simulink model "cart_pendulum_staged_comparison"  (R2018b)
settings: Solver=ode45  StartTime=0.0  StopTime=20  MaxStep=.001  RelTol=1e-8  AbsTol=1e-10
model workspace (MAT data in the model file):
  Ad = [0.884694915571  0.00188314730074  1.9215788783e-06; -2.27514939191  0.997683753616  0.00199844203344; -15.0651784059  -0.0153726310264  0.99998964827]
  Bd = [0.115305084429  1.9215788783e-06; 2.27514939191  0.00199844203344; 15.0651784059  -1.0351730262e-05]
  I = 0.006
  K = [-10 -10.945744415 59.5938842387 10.3435378998]
  M = 0.5
  b = 0.1
  disturbance_ts = [0  0; 8  1; 8.1  0; 20  0]
  g = 9.8
  l = 0.3
  m = 0.2
  z0 = [0; 0; 0.0872664625997; 0]
settings Model: Creator=volka  LastModifiedBy=volka
settings DataIOCC: ReturnWorkspaceOutputs=on

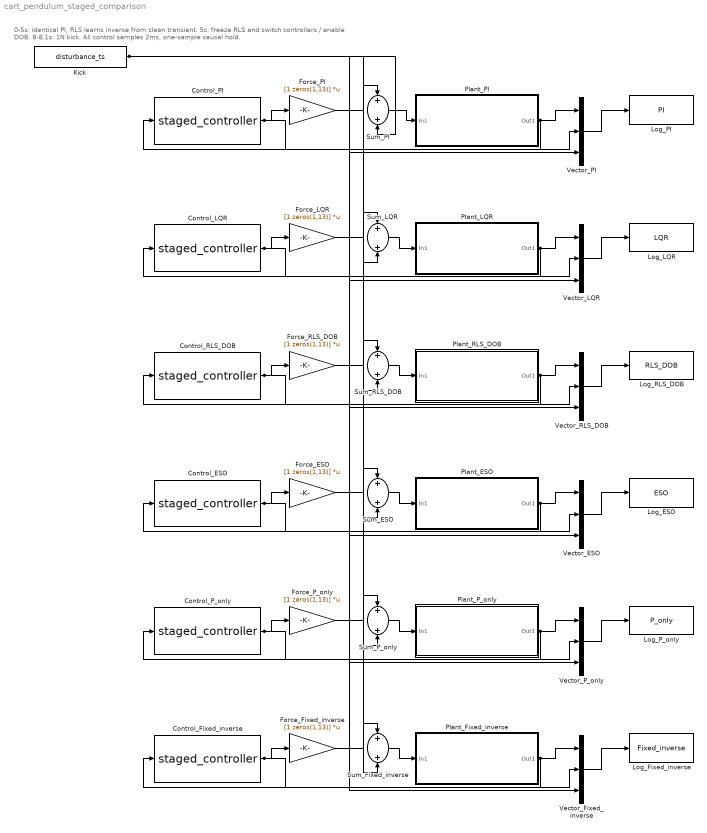
== system cart_pendulum_staged_comparison ==
  note: 0-5s: identical PI, RLS learns inverse from clean transient. 5s: freeze RLS and switch controllers / enable DOB. 8-8.1s: 1N kick. All control samples 2ms, one-sample causal hold.
  Control_ESO : S-Function  FunctionName=staged_controller  Parameters=4,K,Ad,Bd  SFunctionDeploymentMode=off  EnableBusSupport=off
  Control_Fixed_inverse : S-Function  FunctionName=staged_controller  Parameters=6,K,Ad,Bd  SFunctionDeploymentMode=off  EnableBusSupport=off
  Control_LQR : S-Function  FunctionName=staged_controller  Parameters=2,K,Ad,Bd  SFunctionDeploymentMode=off  EnableBusSupport=off
  Control_PI : S-Function  FunctionName=staged_controller  Parameters=1,K,Ad,Bd  SFunctionDeploymentMode=off  EnableBusSupport=off
  Control_P_only : S-Function  FunctionName=staged_controller  Parameters=5,K,Ad,Bd  SFunctionDeploymentMode=off  EnableBusSupport=off
  Control_RLS_DOB : S-Function  FunctionName=staged_controller  Parameters=3,K,Ad,Bd  SFunctionDeploymentMode=off  EnableBusSupport=off
  Force_ESO : Gain  Gain=[1 zeros(1,13)]  Multiplication=Matrix(K*u)
  Force_Fixed_inverse : Gain  Gain=[1 zeros(1,13)]  Multiplication=Matrix(K*u)
  Force_LQR : Gain  Gain=[1 zeros(1,13)]  Multiplication=Matrix(K*u)
  Force_PI : Gain  Gain=[1 zeros(1,13)]  Multiplication=Matrix(K*u)
  Force_P_only : Gain  Gain=[1 zeros(1,13)]  Multiplication=Matrix(K*u)
  Force_RLS_DOB : Gain  Gain=[1 zeros(1,13)]  Multiplication=Matrix(K*u)
  Kick : FromWorkspace  VariableName=disturbance_ts  SampleTime=0  Interpolate=off  OutputAfterFinalValue=Holding final value
  Log_ESO : ToWorkspace  VariableName=ESO  SaveFormat=Structure With Time  SampleTime=-1
  Log_Fixed_inverse : ToWorkspace  VariableName=Fixed_inverse  SaveFormat=Structure With Time  SampleTime=-1
  Log_LQR : ToWorkspace  VariableName=LQR  SaveFormat=Structure With Time  SampleTime=-1
  Log_PI : ToWorkspace  VariableName=PI  SaveFormat=Structure With Time  SampleTime=-1
  Log_P_only : ToWorkspace  VariableName=P_only  SaveFormat=Structure With Time  SampleTime=-1
  Log_RLS_DOB : ToWorkspace  VariableName=RLS_DOB  SaveFormat=Structure With Time  SampleTime=-1
  Plant_ESO : Subsystem
  Plant_Fixed_inverse : Subsystem
  Plant_LQR : Subsystem
  Plant_PI : Subsystem
  Plant_P_only : Subsystem
  Plant_RLS_DOB : Subsystem
  Sum_ESO : Sum
  Sum_Fixed_inverse : Sum
  Sum_LQR : Sum
  Sum_PI : Sum
  Sum_P_only : Sum
  Sum_RLS_DOB : Sum
  Vector_ESO : Mux  Inputs=3
  Vector_Fixed_inverse : Mux  Inputs=3
  Vector_LQR : Mux  Inputs=3
  Vector_PI : Mux  Inputs=3
  Vector_P_only : Mux  Inputs=3
  Vector_RLS_DOB : Mux  Inputs=3
  wires:
  Plant_PI/1(Out1) -> Control_PI/1, Vector_PI/1
  Control_PI/1 -> Force_PI/1, Vector_PI/2
  Force_PI/1 -> Sum_PI/1
  Kick/1 -> Sum_PI/2, Vector_PI/3, Sum_LQR/2, Vector_LQR/3, Sum_RLS_DOB/2, Vector_RLS_DOB/3, Sum_ESO/2, Vector_ESO/3, Sum_P_only/2, Vector_P_only/3, Sum_Fixed_inverse/2, Vector_Fixed_inverse/3
  Sum_PI/1 -> Plant_PI/1(In1)
  Vector_PI/1 -> Log_PI/1
  Plant_LQR/1(Out1) -> Control_LQR/1, Vector_LQR/1
  Control_LQR/1 -> Force_LQR/1, Vector_LQR/2
  Force_LQR/1 -> Sum_LQR/1
  Sum_LQR/1 -> Plant_LQR/1(In1)
  Vector_LQR/1 -> Log_LQR/1
  Plant_RLS_DOB/1(Out1) -> Control_RLS_DOB/1, Vector_RLS_DOB/1
  Control_RLS_DOB/1 -> Force_RLS_DOB/1, Vector_RLS_DOB/2
  Force_RLS_DOB/1 -> Sum_RLS_DOB/1
  Sum_RLS_DOB/1 -> Plant_RLS_DOB/1(In1)
  Vector_RLS_DOB/1 -> Log_RLS_DOB/1
  Plant_ESO/1(Out1) -> Control_ESO/1, Vector_ESO/1
  Control_ESO/1 -> Force_ESO/1, Vector_ESO/2
  Force_ESO/1 -> Sum_ESO/1
  Sum_ESO/1 -> Plant_ESO/1(In1)
  Vector_ESO/1 -> Log_ESO/1
  Plant_P_only/1(Out1) -> Control_P_only/1, Vector_P_only/1
  Control_P_only/1 -> Force_P_only/1, Vector_P_only/2
  Force_P_only/1 -> Sum_P_only/1
  Sum_P_only/1 -> Plant_P_only/1(In1)
  Vector_P_only/1 -> Log_P_only/1
  Plant_Fixed_inverse/1(Out1) -> Control_Fixed_inverse/1, Vector_Fixed_inverse/1
  Control_Fixed_inverse/1 -> Force_Fixed_inverse/1, Vector_Fixed_inverse/2
  Force_Fixed_inverse/1 -> Sum_Fixed_inverse/1
  Sum_Fixed_inverse/1 -> Plant_Fixed_inverse/1(In1)
  Vector_Fixed_inverse/1 -> Log_Fixed_inverse/1

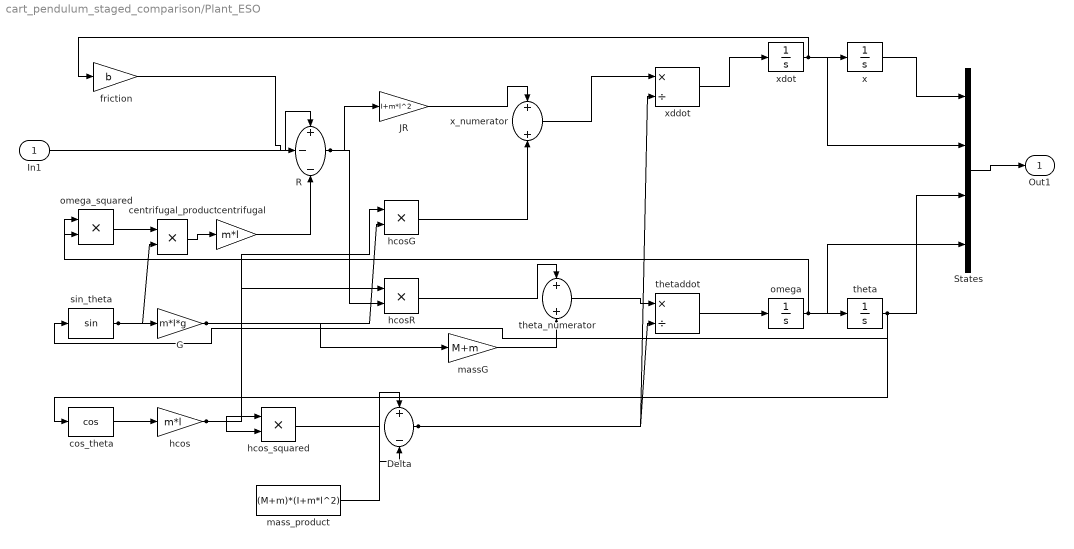
== system cart_pendulum_staged_comparison/Plant_ESO ==
  In1 : Inport
  Delta : Sum  Inputs=+-
  G : Gain  Gain=m*l*g
  JR : Gain  Gain=I+m*l^2
  R : Sum  Inputs=+--
  States : Mux
  centrifugal : Gain  Gain=m*l
  centrifugal_product : Product  Inputs=**
  cos_theta : Trigonometry  Operator=cos
  friction : Gain  Gain=b
  hcos : Gain  Gain=m*l
  hcosG : Product  Inputs=**
  hcosR : Product  Inputs=**
  hcos_squared : Product  Inputs=**
  massG : Gain  Gain=M+m
  mass_product : Constant  Value=(M+m)*(I+m*l^2)
  omega : Integrator  InitialCondition=z0(4)
  omega_squared : Product  Inputs=**
  sin_theta : Trigonometry
  theta : Integrator  InitialCondition=z0(3)
  theta_numerator : Sum
  thetaddot : Product  Inputs=*/
  x : Integrator  InitialCondition=z0(1)
  x_numerator : Sum
  xddot : Product  Inputs=*/
  xdot : Integrator  InitialCondition=z0(2)
  Out1 : Outport
  wires:
  States/1 -> Out1/1
  x/1 -> States/1
  thetaddot/1 -> omega/1
  xddot/1 -> xdot/1
  theta_numerator/1 -> thetaddot/1
  Delta/1 -> thetaddot/2, xddot/2
  x_numerator/1 -> xddot/1
  massG/1 -> theta_numerator/2
  hcosR/1 -> theta_numerator/1
  hcosG/1 -> x_numerator/2
  JR/1 -> x_numerator/1
  G/1 -> massG/1, hcosG/2
  R/1 -> hcosR/2, JR/1
  hcos_squared/1 -> Delta/2
  mass_product/1 -> Delta/1
  hcos/1 -> hcosR/1, hcosG/1, hcos_squared/2, hcos_squared/1
  cos_theta/1 -> hcos/1
  centrifugal/1 -> R/3
  centrifugal_product/1 -> centrifugal/1
  sin_theta/1 -> G/1, centrifugal_product/2
  theta/1 -> States/3, cos_theta/1, sin_theta/1
  omega_squared/1 -> centrifugal_product/1
  omega/1 -> States/4, theta/1, omega_squared/2, omega_squared/1
  friction/1 -> R/2
  xdot/1 -> States/2, x/1, friction/1
  In1/1 -> R/1

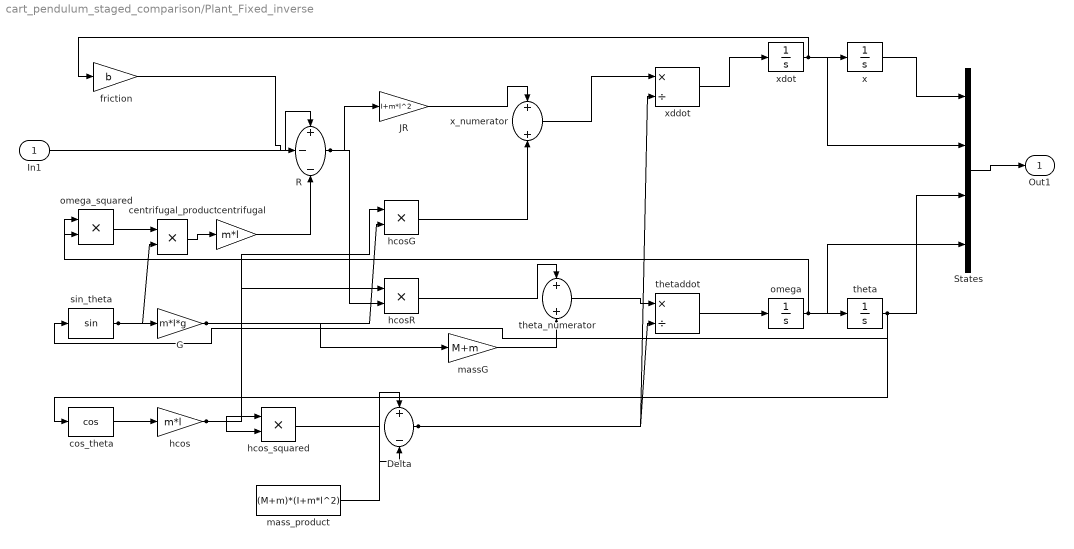
== system cart_pendulum_staged_comparison/Plant_Fixed_inverse ==
  In1 : Inport
  Delta : Sum  Inputs=+-
  G : Gain  Gain=m*l*g
  JR : Gain  Gain=I+m*l^2
  R : Sum  Inputs=+--
  States : Mux
  centrifugal : Gain  Gain=m*l
  centrifugal_product : Product  Inputs=**
  cos_theta : Trigonometry  Operator=cos
  friction : Gain  Gain=b
  hcos : Gain  Gain=m*l
  hcosG : Product  Inputs=**
  hcosR : Product  Inputs=**
  hcos_squared : Product  Inputs=**
  massG : Gain  Gain=M+m
  mass_product : Constant  Value=(M+m)*(I+m*l^2)
  omega : Integrator  InitialCondition=z0(4)
  omega_squared : Product  Inputs=**
  sin_theta : Trigonometry
  theta : Integrator  InitialCondition=z0(3)
  theta_numerator : Sum
  thetaddot : Product  Inputs=*/
  x : Integrator  InitialCondition=z0(1)
  x_numerator : Sum
  xddot : Product  Inputs=*/
  xdot : Integrator  InitialCondition=z0(2)
  Out1 : Outport
  wires:
  States/1 -> Out1/1
  x/1 -> States/1
  thetaddot/1 -> omega/1
  xddot/1 -> xdot/1
  theta_numerator/1 -> thetaddot/1
  Delta/1 -> thetaddot/2, xddot/2
  x_numerator/1 -> xddot/1
  massG/1 -> theta_numerator/2
  hcosR/1 -> theta_numerator/1
  hcosG/1 -> x_numerator/2
  JR/1 -> x_numerator/1
  G/1 -> massG/1, hcosG/2
  R/1 -> hcosR/2, JR/1
  hcos_squared/1 -> Delta/2
  mass_product/1 -> Delta/1
  hcos/1 -> hcosR/1, hcosG/1, hcos_squared/2, hcos_squared/1
  cos_theta/1 -> hcos/1
  centrifugal/1 -> R/3
  centrifugal_product/1 -> centrifugal/1
  sin_theta/1 -> G/1, centrifugal_product/2
  theta/1 -> States/3, cos_theta/1, sin_theta/1
  omega_squared/1 -> centrifugal_product/1
  omega/1 -> States/4, theta/1, omega_squared/2, omega_squared/1
  friction/1 -> R/2
  xdot/1 -> States/2, x/1, friction/1
  In1/1 -> R/1

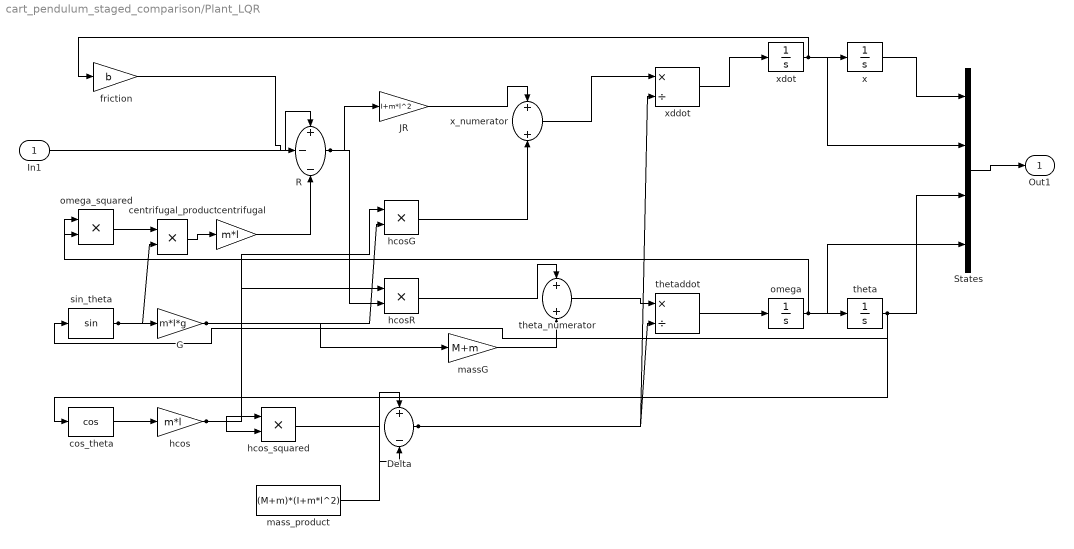
== system cart_pendulum_staged_comparison/Plant_LQR ==
  In1 : Inport
  Delta : Sum  Inputs=+-
  G : Gain  Gain=m*l*g
  JR : Gain  Gain=I+m*l^2
  R : Sum  Inputs=+--
  States : Mux
  centrifugal : Gain  Gain=m*l
  centrifugal_product : Product  Inputs=**
  cos_theta : Trigonometry  Operator=cos
  friction : Gain  Gain=b
  hcos : Gain  Gain=m*l
  hcosG : Product  Inputs=**
  hcosR : Product  Inputs=**
  hcos_squared : Product  Inputs=**
  massG : Gain  Gain=M+m
  mass_product : Constant  Value=(M+m)*(I+m*l^2)
  omega : Integrator  InitialCondition=z0(4)
  omega_squared : Product  Inputs=**
  sin_theta : Trigonometry
  theta : Integrator  InitialCondition=z0(3)
  theta_numerator : Sum
  thetaddot : Product  Inputs=*/
  x : Integrator  InitialCondition=z0(1)
  x_numerator : Sum
  xddot : Product  Inputs=*/
  xdot : Integrator  InitialCondition=z0(2)
  Out1 : Outport
  wires:
  States/1 -> Out1/1
  x/1 -> States/1
  thetaddot/1 -> omega/1
  xddot/1 -> xdot/1
  theta_numerator/1 -> thetaddot/1
  Delta/1 -> thetaddot/2, xddot/2
  x_numerator/1 -> xddot/1
  massG/1 -> theta_numerator/2
  hcosR/1 -> theta_numerator/1
  hcosG/1 -> x_numerator/2
  JR/1 -> x_numerator/1
  G/1 -> massG/1, hcosG/2
  R/1 -> hcosR/2, JR/1
  hcos_squared/1 -> Delta/2
  mass_product/1 -> Delta/1
  hcos/1 -> hcosR/1, hcosG/1, hcos_squared/2, hcos_squared/1
  cos_theta/1 -> hcos/1
  centrifugal/1 -> R/3
  centrifugal_product/1 -> centrifugal/1
  sin_theta/1 -> G/1, centrifugal_product/2
  theta/1 -> States/3, cos_theta/1, sin_theta/1
  omega_squared/1 -> centrifugal_product/1
  omega/1 -> States/4, theta/1, omega_squared/2, omega_squared/1
  friction/1 -> R/2
  xdot/1 -> States/2, x/1, friction/1
  In1/1 -> R/1

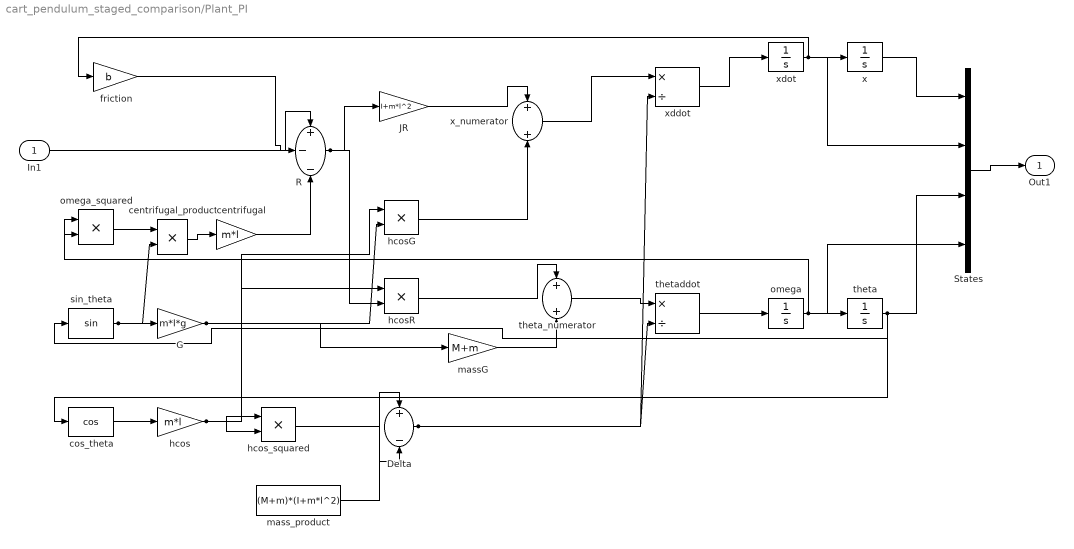
== system cart_pendulum_staged_comparison/Plant_PI ==
  In1 : Inport
  Delta : Sum  Inputs=+-
  G : Gain  Gain=m*l*g
  JR : Gain  Gain=I+m*l^2
  R : Sum  Inputs=+--
  States : Mux
  centrifugal : Gain  Gain=m*l
  centrifugal_product : Product  Inputs=**
  cos_theta : Trigonometry  Operator=cos
  friction : Gain  Gain=b
  hcos : Gain  Gain=m*l
  hcosG : Product  Inputs=**
  hcosR : Product  Inputs=**
  hcos_squared : Product  Inputs=**
  massG : Gain  Gain=M+m
  mass_product : Constant  Value=(M+m)*(I+m*l^2)
  omega : Integrator  InitialCondition=z0(4)
  omega_squared : Product  Inputs=**
  sin_theta : Trigonometry
  theta : Integrator  InitialCondition=z0(3)
  theta_numerator : Sum
  thetaddot : Product  Inputs=*/
  x : Integrator  InitialCondition=z0(1)
  x_numerator : Sum
  xddot : Product  Inputs=*/
  xdot : Integrator  InitialCondition=z0(2)
  Out1 : Outport
  wires:
  States/1 -> Out1/1
  x/1 -> States/1
  thetaddot/1 -> omega/1
  xddot/1 -> xdot/1
  theta_numerator/1 -> thetaddot/1
  Delta/1 -> thetaddot/2, xddot/2
  x_numerator/1 -> xddot/1
  massG/1 -> theta_numerator/2
  hcosR/1 -> theta_numerator/1
  hcosG/1 -> x_numerator/2
  JR/1 -> x_numerator/1
  G/1 -> massG/1, hcosG/2
  R/1 -> hcosR/2, JR/1
  hcos_squared/1 -> Delta/2
  mass_product/1 -> Delta/1
  hcos/1 -> hcosR/1, hcosG/1, hcos_squared/2, hcos_squared/1
  cos_theta/1 -> hcos/1
  centrifugal/1 -> R/3
  centrifugal_product/1 -> centrifugal/1
  sin_theta/1 -> G/1, centrifugal_product/2
  theta/1 -> States/3, cos_theta/1, sin_theta/1
  omega_squared/1 -> centrifugal_product/1
  omega/1 -> States/4, theta/1, omega_squared/2, omega_squared/1
  friction/1 -> R/2
  xdot/1 -> States/2, x/1, friction/1
  In1/1 -> R/1

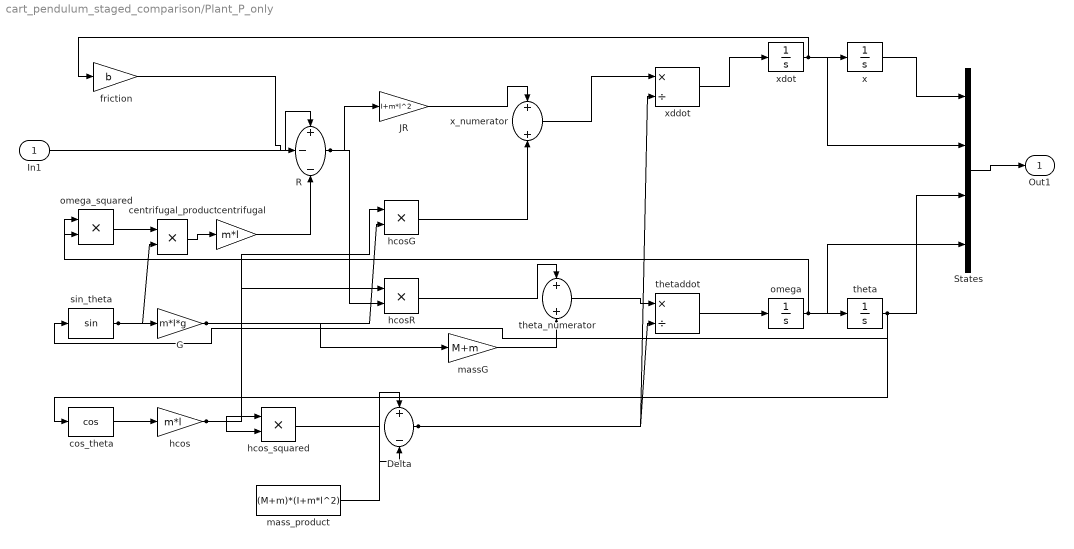
== system cart_pendulum_staged_comparison/Plant_P_only ==
  In1 : Inport
  Delta : Sum  Inputs=+-
  G : Gain  Gain=m*l*g
  JR : Gain  Gain=I+m*l^2
  R : Sum  Inputs=+--
  States : Mux
  centrifugal : Gain  Gain=m*l
  centrifugal_product : Product  Inputs=**
  cos_theta : Trigonometry  Operator=cos
  friction : Gain  Gain=b
  hcos : Gain  Gain=m*l
  hcosG : Product  Inputs=**
  hcosR : Product  Inputs=**
  hcos_squared : Product  Inputs=**
  massG : Gain  Gain=M+m
  mass_product : Constant  Value=(M+m)*(I+m*l^2)
  omega : Integrator  InitialCondition=z0(4)
  omega_squared : Product  Inputs=**
  sin_theta : Trigonometry
  theta : Integrator  InitialCondition=z0(3)
  theta_numerator : Sum
  thetaddot : Product  Inputs=*/
  x : Integrator  InitialCondition=z0(1)
  x_numerator : Sum
  xddot : Product  Inputs=*/
  xdot : Integrator  InitialCondition=z0(2)
  Out1 : Outport
  wires:
  States/1 -> Out1/1
  x/1 -> States/1
  thetaddot/1 -> omega/1
  xddot/1 -> xdot/1
  theta_numerator/1 -> thetaddot/1
  Delta/1 -> thetaddot/2, xddot/2
  x_numerator/1 -> xddot/1
  massG/1 -> theta_numerator/2
  hcosR/1 -> theta_numerator/1
  hcosG/1 -> x_numerator/2
  JR/1 -> x_numerator/1
  G/1 -> massG/1, hcosG/2
  R/1 -> hcosR/2, JR/1
  hcos_squared/1 -> Delta/2
  mass_product/1 -> Delta/1
  hcos/1 -> hcosR/1, hcosG/1, hcos_squared/2, hcos_squared/1
  cos_theta/1 -> hcos/1
  centrifugal/1 -> R/3
  centrifugal_product/1 -> centrifugal/1
  sin_theta/1 -> G/1, centrifugal_product/2
  theta/1 -> States/3, cos_theta/1, sin_theta/1
  omega_squared/1 -> centrifugal_product/1
  omega/1 -> States/4, theta/1, omega_squared/2, omega_squared/1
  friction/1 -> R/2
  xdot/1 -> States/2, x/1, friction/1
  In1/1 -> R/1

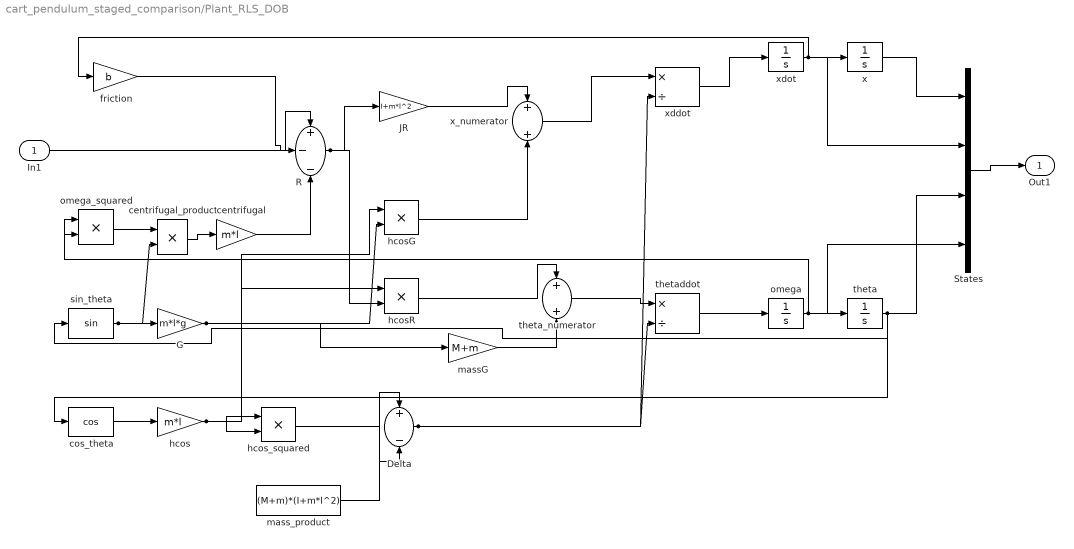
== system cart_pendulum_staged_comparison/Plant_RLS_DOB ==
  In1 : Inport
  Delta : Sum  Inputs=+-
  G : Gain  Gain=m*l*g
  JR : Gain  Gain=I+m*l^2
  R : Sum  Inputs=+--
  States : Mux
  centrifugal : Gain  Gain=m*l
  centrifugal_product : Product  Inputs=**
  cos_theta : Trigonometry  Operator=cos
  friction : Gain  Gain=b
  hcos : Gain  Gain=m*l
  hcosG : Product  Inputs=**
  hcosR : Product  Inputs=**
  hcos_squared : Product  Inputs=**
  massG : Gain  Gain=M+m
  mass_product : Constant  Value=(M+m)*(I+m*l^2)
  omega : Integrator  InitialCondition=z0(4)
  omega_squared : Product  Inputs=**
  sin_theta : Trigonometry
  theta : Integrator  InitialCondition=z0(3)
  theta_numerator : Sum
  thetaddot : Product  Inputs=*/
  x : Integrator  InitialCondition=z0(1)
  x_numerator : Sum
  xddot : Product  Inputs=*/
  xdot : Integrator  InitialCondition=z0(2)
  Out1 : Outport
  wires:
  States/1 -> Out1/1
  x/1 -> States/1
  thetaddot/1 -> omega/1
  xddot/1 -> xdot/1
  theta_numerator/1 -> thetaddot/1
  Delta/1 -> thetaddot/2, xddot/2
  x_numerator/1 -> xddot/1
  massG/1 -> theta_numerator/2
  hcosR/1 -> theta_numerator/1
  hcosG/1 -> x_numerator/2
  JR/1 -> x_numerator/1
  G/1 -> massG/1, hcosG/2
  R/1 -> hcosR/2, JR/1
  hcos_squared/1 -> Delta/2
  mass_product/1 -> Delta/1
  hcos/1 -> hcosR/1, hcosG/1, hcos_squared/2, hcos_squared/1
  cos_theta/1 -> hcos/1
  centrifugal/1 -> R/3
  centrifugal_product/1 -> centrifugal/1
  sin_theta/1 -> G/1, centrifugal_product/2
  theta/1 -> States/3, cos_theta/1, sin_theta/1
  omega_squared/1 -> centrifugal_product/1
  omega/1 -> States/4, theta/1, omega_squared/2, omega_squared/1
  friction/1 -> R/2
  xdot/1 -> States/2, x/1, friction/1
  In1/1 -> R/1
